simulink model "task6_model"  (R2014b)
settings: Solver=ode45  StartTime=0.0  StopTime=3  RelTol=1e-3
values from neighbouring files (symbols this model uses):
  A = [-(R/L) -(kE/L) ; kM/J -(Cv/J)]    [create_ss.m]    (also in task6.m = [0 0 1 0; 0 0 0 1; -kt/Jtot kt*n^2/Jtot -dt/Jtot dt*n^2/Jtot)
  B = [1/L ; 0]    [create_ss.m]    (also in task6.m = [0; 0; 1/Jtot ; 0])
  C = [0 1]    [create_ss.m]    (also in task6.m = eye(4))
  Cv = 1.3*10^(-3) *10^(-3)*60/(2*pi)    (= 1.24140855612e-05)    [load_values.m]    (also in task6.m)
  D = zeros(size(B))    [task6.m]
  J = 60 * 10^(-3) *10^(-4)    (= 6e-06)    [load_values.m]    (also in task6.m)
  kE = 4.555 *10^(-3)*60/(2*pi)    (= 0.043497045947)    [load_values.m]    (also in task6.m)
  kM = 43.5*10^(-3)    (= 0.0435)    [load_values.m]    (also in task6.m)
  L = [24.5, 19.6, 13.9, 13.1, 7   ] *10^(-3)    [load_values.m]    (also in task6.m = 0.00011)
  R = 1.45    [load_values.m]    (also in task6.m)
settings Model: Creator=davidebo  LastModifiedBy=davidebo

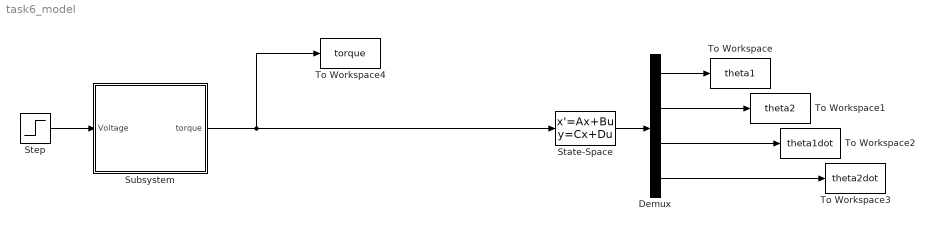
== system task6_model ==
  Demux : Demux
  State-Space : StateSpace  A=A  B=B  C=C  D=D  X0=0
  Step : Step  SampleTime=0
  Subsystem : Subsystem
  To Workspace : ToWorkspace  VariableName=theta1  SaveFormat=Timeseries  SampleTime=-1
  To Workspace1 : ToWorkspace  VariableName=theta2  SaveFormat=Timeseries  SampleTime=-1
  To Workspace2 : ToWorkspace  VariableName=theta1dot  SaveFormat=Timeseries  SampleTime=-1
  To Workspace3 : ToWorkspace  VariableName=theta2dot  SaveFormat=Timeseries  SampleTime=-1
  To Workspace4 : ToWorkspace  VariableName=torque  SaveFormat=Timeseries  SampleTime=-1
  wires:
  State-Space/1 -> Demux/1
  Subsystem/1(torque) -> To Workspace4/1, State-Space/1
  Demux/1 -> To Workspace/1
  Demux/2 -> To Workspace1/1
  Demux/3 -> To Workspace2/1
  Demux/4 -> To Workspace3/1
  Step/1 -> Subsystem/1(Voltage)

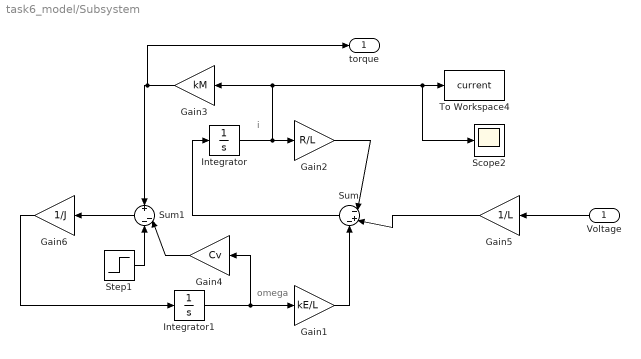
== system task6_model/Subsystem ==
  note: omega
  note: i
  Voltage : Inport
  Gain1 : Gain  Gain=kE/L
  Gain2 : Gain  Gain=R/L
  Gain3 : Gain  Gain=kM
  Gain4 : Gain  Gain=Cv
  Gain5 : Gain  Gain=1/L
  Gain6 : Gain  Gain=1/J
  Integrator : Integrator
  Integrator1 : Integrator
  Scope2 : Scope
      settings: TimeRange=10  SaveName=ScopeData3
  Step1 : Step  Time=2  After=0  SampleTime=0
  Sum : Sum  Inputs=|-+-
  Sum1 : Sum  Inputs=+|--
  To Workspace4 : ToWorkspace  VariableName=current  SaveFormat=Timeseries  SampleTime=-1
  torque : Outport
  wires:
  Gain5/1 -> Sum/2
  Integrator1/1 -> Gain4/1, Gain1/1
  Gain2/1 -> Sum/1
  Sum1/1 -> Gain6/1
  Gain1/1 -> Sum/3
  Voltage/1 -> Gain5/1
  Gain3/1 -> torque/1, Sum1/1
  Step1/1 -> Sum1/3
  Gain4/1 -> Sum1/2
  Gain6/1 -> Integrator1/1
  Integrator/1 -> Scope2/1, To Workspace4/1, Gain3/1, Gain2/1
  Sum/1 -> Integrator/1
